simulink model "TP3_4"  (R2018a)
settings: Solver=ode45  StartTime=0.0  StopTime=10.0  RelTol=1e-3
libraries: dsparch4 x5, commsynccomp2 x2, commrflib2 x1
settings Model: Creator=10RS6N  LastModifiedBy=10RS5
settings DataIOCC: SaveFormat=StructureWithTime  ReturnWorkspaceOutputs=on
settings OptimizationCC: LifeSpan=inf
settings DebuggingCC: SFExecutionAtInitializationDiag=none
settings HardwareCC: ProdBitPerSizeT=32  ProdBitPerPtrDiffT=32  ProdWordSize=32  ProdHWDeviceType=Specified
settings SFSimCC: SimUseLocalCustomCode=on
settings RTWCC: RTWUseLocalCustomCode=on
settings CodeAppCC: StateflowObjectComments=on

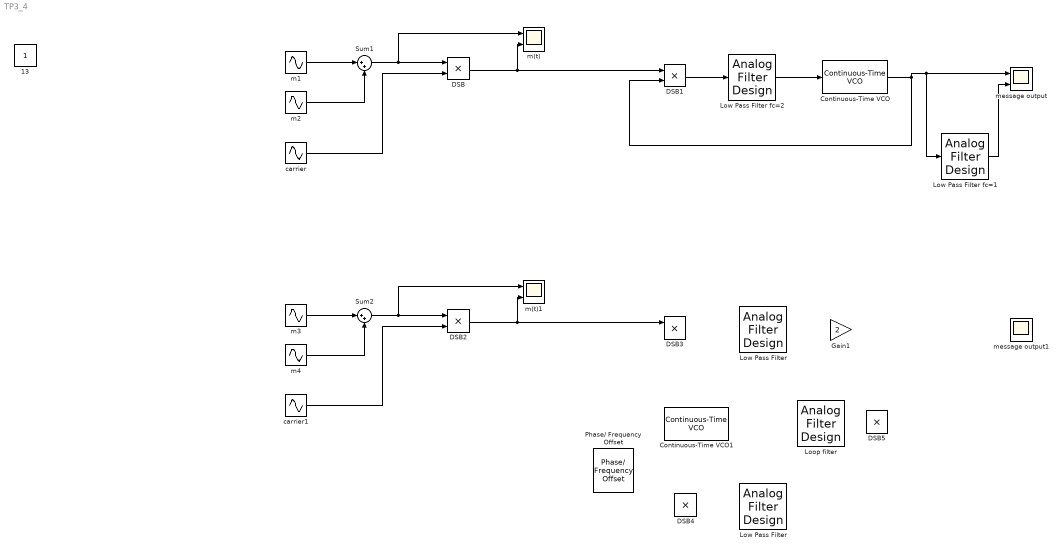
== system TP3_4 ==
  Continuous-Time VCO : commsynccomp2/Continuous-Time VCO  Ac=1  Fc=30  Kc=1  Ph=pi/4
      settings: SourceProductName=Communications System Toolbox  SourceProductBaseCode=CM
  Continuous-Time VCO1 : commsynccomp2/Continuous-Time VCO  Ac=1  Fc=10  Kc=1  Ph=pi/4
      settings: SourceProductName=Communications System Toolbox  SourceProductBaseCode=CM
  DSB{,1..5} (6 alike) : Product
  Gain1 : Gain  Gain=2
  Loop filter : dsparch4/Analog Filter Design  method=Butterworth  filttype=Lowpass  N=10  Wlo=50*2*pi  Whi=1319.46  Rp=2  Rs=40
  Low Pass Filter : dsparch4/Analog Filter Design  method=Butterworth  filttype=Lowpass  N=10  Wlo=50*2*pi  Whi=1319.46  Rp=2  Rs=40
  Low Pass Filter fc=1 : dsparch4/Analog Filter Design  method=Butterworth  filttype=Lowpass  N=10  Wlo=13*2*pi  Whi=1319.46  Rp=2  Rs=40
  Low Pass Filter fc=2 : dsparch4/Analog Filter Design  method=Butterworth  filttype=Lowpass  N=10  Wlo=33*2*pi  Whi=1319.46  Rp=2  Rs=40
  "Low Pass Filter " : dsparch4/Analog Filter Design  method=Butterworth  filttype=Lowpass  N=10  Wlo=50*2*pi  Whi=1319.46  Rp=2  Rs=40
  Phase/ Frequency Offset : commrflib2/Phase// Frequency Offset  phaseOffset=pi/2  freqPort=off  freqOffset=0
      settings: SourceProductName=Communications System Toolbox
  Sum1 : Sum  Inputs=|++
  Sum2 : Sum  Inputs=|++
  carrier : Sin  Frequency=500*2*pi  SampleTime=0
  carrier1 : Sin  Frequency=500*2*pi  SampleTime=0
  m(t) : Scope  NumInputPorts=2
  m(t)1 : Scope  NumInputPorts=2
  m1 : Sin  Frequency=5*2*pi  SampleTime=0
  m2 : Sin  Amplitude=0.5  Frequency=10*2*pi  SampleTime=0
  m3 : Sin  Frequency=5*2*pi  SampleTime=0
  m4 : Sin  Amplitude=0.5  Frequency=10*2*pi  SampleTime=0
  message output : Scope  NumInputPorts=2
  message output1 : Scope
  13 : Constant  IOType=siggen
  wires:
  m1/1 -> Sum1/1
  m2/1 -> Sum1/2
  Sum1/1 -> m(t)/1, DSB/1
  carrier/1 -> DSB/2
  DSB/1 -> DSB1/1, m(t)/2
  DSB1/1 -> Low Pass Filter fc=2/1
  carrier1/1 -> DSB2/2
  Sum2/1 -> DSB2/1, m(t)1/1
  m4/1 -> Sum2/2
  m3/1 -> Sum2/1
  DSB2/1 -> m(t)1/2, DSB3/1
  Low Pass Filter fc=1/1 -> message output/2
  Low Pass Filter fc=2/1 -> Continuous-Time VCO/1
  Continuous-Time VCO/1 -> DSB1/2, Low Pass Filter fc=1/1, message output/1
